simulink model "Car_15_Jan_addtimerrelay_2012b"  (Simulink 8.0)
settings: Solver=ode5  StartTime=0.0  StopTime=inf  FixedStep=sample_time  RelTol=1e-3
InitFcn:
  | sample_time=0.005;%0.004;%0.0025;%0.02;
  | sample_time_Vicon = 0.005;
  | DeltaT = 0.02;
  | g = 9.81;
  | H0 = g%0.3165;
  | Kl = 1;
  | 
  | Q6_mass = 0.84;
  | 
  | Q6_Omega_r = 1.5; %for horizon ref
  | Q6_Zeta_r = 0.5; %for horizon ref
  | Q6_Omega_r_h = 2;%for vertical ref
  | Q6_Zeta_r_h = 2; %for vertical ref
  | 
  | 
  | Q6_Omega = 1.5; %for horizon control
  | Q6_Zeta = 0.5; %for horizon control
  | Q6_Omega_h= 2; %for vertical control
  | Q6_Zeta_h = 0.7; %for vertical control
  | 
  | 
  | Q6_acc_max = 5;%horizontal max acc
  | Q6_acc_max_h = 3;%horizontal max acc
  | 
  | omega_circle = 72*pi/180;
  | omega_h = 0.1;%Ascending speed
  | PI = pi;
  | Circle_R = 2.5;
  | MAX_Height = -2;
undefined symbols (not defined in the file or in its folder): DiscIntNeverNeededParam, serial
libraries: simulink x9, dspswit3 x5, X330_Control x4, instrumentlib x2
(part 2 of 2)

== stateflow chart UAV 1/Trajectory Logic/stateflowforwholesequence ==
  state Landing
    state Decsending
      en:smooth_flag = 1;pwm = 1850;
      du:PosDesired[2] = (landing_area[2] - PosDesired[2])*1*DeltaT + PosDesired[2] ;
    state CutThrottle
      du:HoverThrottle = (0.0 - HoverThrottle)*2*DeltaT + HoverThrottle ;
    (default) -> Decsending : {PosDesired = Pos;smooth_flag = 1;relay = 1;}
    Decsending -> CutThrottle : [Pos[2] > landing_area[2]-0.05]
  state Airborne1
    state TakeOff
      du:HoverThrottle = (H0 - HoverThrottle)*2*DeltaT + HoverThrottle ;
    state capturing_sequence
      state caputuring_test1
        en: PosDesired = Pos; PosDesired[2] = -1.3;smooth_flag = 1;
      state hoverstate
        en:PosDesired = Pos;PosDesired[2] = -1.3;pwm = 1450;
      state move_origin5
        du:PosDesired[1] = (ly - PosDesired[1])*1*DeltaT + PosDesired[1] ;
        PosDesired[0] = lx;
        PosDesired[2] = -1.3
      state move_origin6
        du:PosDesired[1] = 0;
        PosDesired[0] = (lx - PosDesired[0])*1*DeltaT + PosDesired[0] ;
        PosDesired[2] = -1.3
      state move_origin7
        du:PosDesired[1] = (0 - PosDesired[1])*1*DeltaT + PosDesired[1] ;
        PosDesired[0] = (0 - PosDesired[0])*1*DeltaT + PosDesired[0] ;
        PosDesired[2] = -1.3
      state capturing_sequence1
        state capturing_sequence2
          state normal_capturing2
            en: PosDesired[0] = car[0] ; PosDesired[1] = car[1]; PosDesired[2] = -0.5;pwm = 1250;
          state caputuring_test
            en: PosDesired = Pos; PosDesired[2] = -1.3;pwm = 1450;relay = 0;
          state normal_capturing1
            en: PosDesired[0] = carest[0] + 0.3*(car[0] - Pos[0])/abs(car[0] - Pos[0]); PosDesired[1] = carest[1] + 0.3*(car[1] - Pos[1])/(abs(car[1] - Pos[1])); PosDesired[2] = -0.5;pwm = 1650;
          (default) -> normal_capturing1
          normal_capturing2 -> normal_capturing1 [order 1] : after(1,sec)
              | [match_flag ~=1]
          normal_capturing1 -> normal_capturing2 [order 1] : after(1,sec)
              | [match_flag~=1]
          normal_capturing1 -> caputuring_test [order 2] : [match_flag==1]
          caputuring_test -> normal_capturing2 : [match_flag~=1]
          normal_capturing2 -> caputuring_test [order 2] : [match_flag==1]
        (default) -> capturing_sequence2 : {PosDesired = Pos;smooth_flag = 0;pwm = 2100;timerenable = 1;}
      (default) -> capturing_sequence1
      capturing_sequence1 -> caputuring_test1 [order 1] : after(40,sec)
          | [match_flag~=1]
      capturing_sequence1 -> caputuring_test1 [order 2] : [car[2]<-0.4]
      capturing_sequence1 -> caputuring_test1 [order 3] : [RC[5] < 0]
      caputuring_test1 -> (junction 121) : [abs(Pos[2]+1.3)<0.2]
      (junction 121) -> move_origin7 [order 1] : [car[2]>-0.4]
          | {pwm = 1350;}
      (junction 121) -> move_origin7 [order 3] : [RC[5]<0]
          | {pwm = 2100;}
      (junction 121) -> move_origin7 [order 2] : [car[2]<-0.4]
          | {pwm = 1550;}
      move_origin7 -> move_origin6 : [(abs(0 - Pos[1])+abs(0 - Pos[1]))<0.15]
      move_origin6 -> move_origin5 : [(abs(lx - Pos[0])+abs(0-Pos[1]))<0.1]
      move_origin5 -> hoverstate : [(abs(lx - Pos[0])+abs(ly - Pos[1]))<0.1]
    state Hover
      en: PosDesired[2] = -1.3;
    state move_origin1
      du:PosDesired[0] = (0 - PosDesired[0])*1*DeltaT + PosDesired[0] ;PosDesired[1] = 0;
      PosDesired[2] = -1.3
    state Hover1
      en: PosDesired[2] = -1.3;pwm = 1450;
    state move_origin
      du:PosDesired[1] = (0 - PosDesired[1])*1*DeltaT + PosDesired[1] ;PosDesired[0] = landing_area[0];
      PosDesired[2] = -1.3
    (default) -> TakeOff : {PosDesired = Pos;PosDesired[2] = -1.3;smooth_flag = 1;pwm = 1650;lx = Pos[0];ly = Pos[1];relay = 1;timerenable = 0;}
    TakeOff -> Hover : after(5,sec)
    Hover -> move_origin : after(5,sec)
    move_origin -> move_origin1 : after(5,sec)
    move_origin1 -> Hover1 : [(abs(0 - Pos[0])+abs(0 - Pos[1]))<0.2]
        | {PosDesired = Pos;}
    Hover1 -> capturing_sequence : [RC[5] > 0]
  Landing -> Airborne1 : [RC[6] > 0.5]
  Airborne1 -> Landing : [RC[6] < -0.5]
  (default) -> Landing : {HoverThrottle=0.01;}
  data: PosDesired output double size=4; HoverThrottle output double size=1; RC input double size=8; Pos input double size=4; DeltaT parameter double size=1; H0 parameter double size=1; Kl parameter double size=1; VelCmd local double size=2 =0; line_count local int8 size=1 =0; triangle_count local int8 size=1 =0; T_line local double size=1; omega_circle parameter double size=1; PI parameter double size=1; omega_h parameter double; Circle_R parameter double size=1; MAX_Height parameter double size=1; landing_area input double size=6; car input double size=12; carest input double size=2; match_flag input double; smooth_flag output boolean =0; matchx local double; matchy local double; pwm output double; lx local double; ly local double; pwm1 local double; relay output double; timerenable output double; zero input double
